simulink model "InvertedPD"  (Simulink 5.0)
settings: Solver=ode1  SolverMode=SingleTasking  StartTime=0.0  StopTime=70.0  FixedStep=0.001  RelTol=1e-3
libraries: pci1711 x3
CloseFcn:
  | rtwprivate ssgencode ModelCloseRequest InvertedPD
settings Model: LastModifiedBy=AD  ExtModeMexFile=rtwinext  ExtModeTrigMode=oneshot  ExtModeTrigDuration=100000  ExtModeLogAll=off  SimulationMode=external  LimitDataPoints=off  BlockReductionOpt=off  BooleanDataType=off  RTWSystemTargetFile=rtwinfbk.tlc  RTWTemplateMakefile=winfbktmf  RTWOptions="-aCCOptimize=1 -aEnforceIntegerDowncast=1 -aExtMode=1 -aFoldNonRolledExpr=1 -aForceParamTrailComments=0 -aGenerateComments=1 -aGenerateReport=0 -aIncDataTypeInIds=0 -aIncHierarchyInIds=0 -aInlineInvariantSignals=0 -aInlineParameters=0 -aInlinedPrmAccess=\"Literals\" -aLocalBlockOutputs=1 -aMaxRTWIdLen=31 -aPrefixModelToSubsysFcnNames=1 -aRTWVerbose=1 -aRebuildAll=0 -aRollThreshold=5 -aShowEliminatedStatements=1"

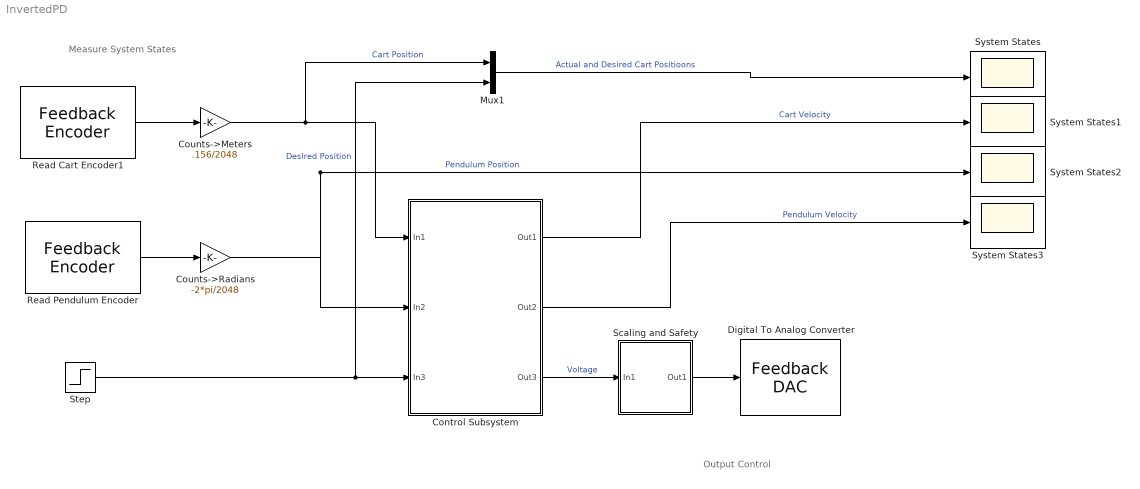
== system InvertedPD ==
  note: Measure System States
  note: Output Control
  Control Subsystem : Subsystem
  Counts->Meters : Gain  Gain=.156/2048  SaturateOnIntegerOverflow=on
  Counts->Radians : Gain  Gain=-2*pi/2048  SaturateOnIntegerOverflow=on
  Digital To Analog Converter : pci1711/Advantech  PCI1711 I//O Board Lib/Feedback DAC  channel=0  range=0  tsamp=0.001  hwAccess=on
  Mux1 : Mux  Inputs=2
  Read Cart Encoder1 : pci1711/Advantech  PCI1711 I//O Board Lib/Feedback Encoder   channel=0  offset=0  tsamp=0.001  hwAccess=on
  Read Pendulum Encoder : pci1711/Advantech  PCI1711 I//O Board Lib/Feedback Encoder   channel=1  offset=-1024  tsamp=0.001  hwAccess=on
  Scaling and Safety : Subsystem
  Step : Step  Time=20  After=0.2  SampleTime=0
  System States{,1..3} (4 alike) : Scope
      System States settings: TimeRange=50  YMin=-0.125  YMax=0.025  SaveName=y  Decimation=0.1  SampleInput=on  SampleTime=0.01
      System States1 settings: TimeRange=50  YMin=-0.125  YMax=0.025  SaveName=y1  Decimation=0.1  SampleInput=on  SampleTime=0.01
      System States2 settings: TimeRange=50  YMin=-0.125  YMax=0.025  SaveName=y2  Decimation=0.1  SampleInput=on  SampleTime=0.01
      System States3 settings: TimeRange=50  YMin=-0.125  YMax=0.025  SaveName=y3  Decimation=0.1  SampleInput=on  SampleTime=0.01
  wires:
  Counts->Meters/1 -> Mux1/1, Control Subsystem/1(In1)  "Cart Position"
  Counts->Radians/1 -> Control Subsystem/2(In2), System States2/1  "Pendulum Position"
  Scaling and Safety/1(Out1) -> Digital To Analog Converter/1
  Step/1 -> Mux1/2, Control Subsystem/3(In3)  "Desired Position"
  Control Subsystem/3(Out3) -> Scaling and Safety/1(In1)  "Voltage"
  Mux1/1 -> System States/1  "Actual and Desired Cart Positioons"
  Read Cart Encoder1/1 -> Counts->Meters/1
  Read Pendulum Encoder/1 -> Counts->Radians/1
  Control Subsystem/1(Out1) -> System States1/1  "Cart Velocity"
  Control Subsystem/2(Out2) -> System States3/1  "Pendulum Velocity"

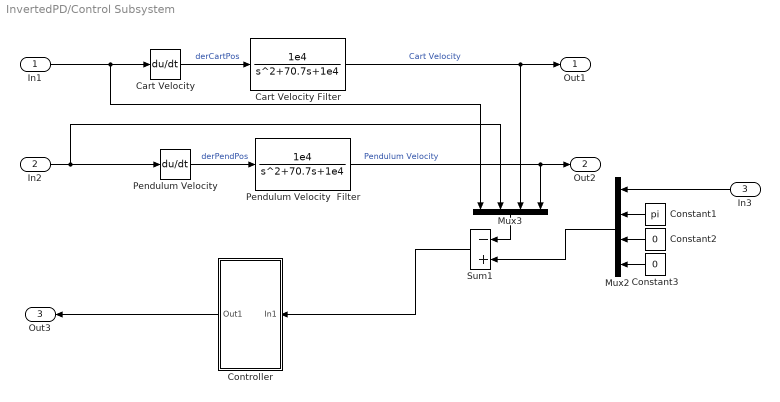
== system InvertedPD/Control Subsystem ==
  In1 : Inport
  In2 : Inport  Port=2
  In3 : Inport  Orientation=left  Port=3
  Cart Velocity : Derivative
  Cart Velocity Filter : TransferFcn  Numerator=[1e4]  Denominator=[1 70.7 1e4]
  Constant1 : Constant  Orientation=left  Value=pi
  Constant2 : Constant  Orientation=left  Value=0
  Constant3 : Constant  Orientation=left  Value=0
  Controller : Subsystem  Orientation=left
  Mux2 : Mux  Orientation=left
  Mux3 : Mux  Orientation=down
  Pendulum Velocity : Derivative
  Pendulum Velocity  Filter : TransferFcn  Numerator=[1e4]  Denominator=[1 70.7 1e4]
  Sum1 : Sum  Orientation=left  Inputs=-+  SaturateOnIntegerOverflow=on  InputSameDT=on
  Out1 : Outport
  Out2 : Outport  Port=2
  Out3 : Outport  Orientation=left  Port=3
  wires:
  Cart Velocity/1 -> Cart Velocity Filter/1  "derCartPos"
  Pendulum Velocity/1 -> Pendulum Velocity  Filter/1  "derPendPos"
  Cart Velocity Filter/1 -> Mux3/3, Out1/1  "Cart Velocity"
  Pendulum Velocity  Filter/1 -> Mux3/4, Out2/1  "Pendulum Velocity"
  Mux2/1 -> Sum1/2
  Constant1/1 -> Mux2/2
  Constant2/1 -> Mux2/3
  Constant3/1 -> Mux2/4
  Mux3/1 -> Sum1/1
  In1/1 -> Cart Velocity/1, Mux3/1
  In2/1 -> Pendulum Velocity/1, Mux3/2
  In3/1 -> Mux2/1
  Controller/1(Out1) -> Out3/1
  Sum1/1 -> Controller/1(In1)

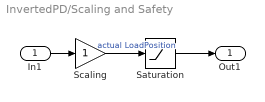
== system InvertedPD/Scaling and Safety ==
  In1 : Inport
  Saturation : Saturate  UpperLimit=2.5  LowerLimit=-2.5
  Scaling : Gain  SaturateOnIntegerOverflow=on
  Out1 : Outport
  wires:
  Saturation/1 -> Out1/1
  In1/1 -> Scaling/1
  Scaling/1 -> Saturation/1  "actual LoadPosition"

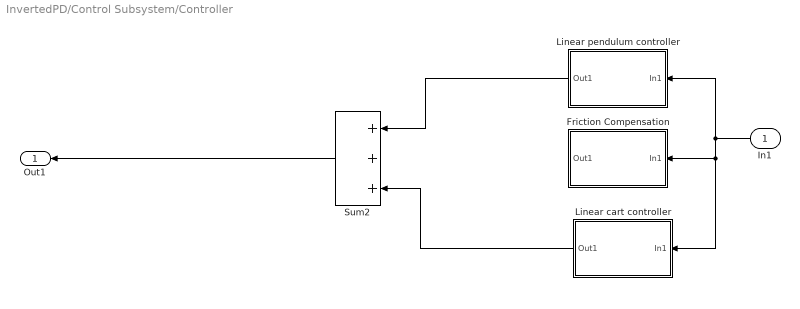
== system InvertedPD/Control Subsystem/Controller ==
  In1 : Inport  Orientation=left
  Friction Compensation : Subsystem  Orientation=left  mask(linear){frictionCompNeg=.1, frictionCompPos=.1}
      mask prompts: frictionCompNeg "Friction Compensation Magnitude in Negative Direction"; frictionCompPos "Friction Compensation Magnitude in Positive Direction"
      mask Display: plot(0,0,100,100,[40,30,20],[87,85,80],[46,54,54,46,46],[90,90,80,80,90],[46,45,45,46,54,55,55,54,46],[78,80,90,91,91,90,80,78,78],[51,51,49,49],[78,10,10,78],[90,80,70,60],[70,80,85,88],[20,10],[80,70],[20,20,15],[73,80,80],[85,80,80],[80,80,74])
  Linear cart controller : Subsystem  Orientation=left  mask(linear){K1=-40, K3=-80}
      mask prompts: K1 "K1  - position  feedback"; K3 "K3  -  velocity  feedback"
      mask Display: plot(0,0,100,100,[40,30,20],[87,85,80],[46,54,54,46,46],[90,90,80,80,90],[46,45,45,46,54,55,55,54,46],[78,80,90,91,91,90,80,78,78],[51,51,49,49],[78,10,10,78],[90,80,70,60],[70,80,85,88],[20,10],[80,70],[20,20,15],[73,80,80],[85,80,80],[80,80,74])
  Linear pendulum controller : Subsystem  Orientation=left  mask(linear){K2=130, K4=35}
      mask prompts: K2 "K2  - angle  feedback"; K4 "K4  - angular velocity  feedback"
      mask Display: plot(0,0,100,100,[40,30,20],[87,85,80],[46,54,54,46,46],[90,90,80,80,90],[46,45,45,46,54,55,55,54,46],[78,80,90,91,91,90,80,78,78],[51,51,49,49],[78,10,10,78],[90,80,70,60],[70,80,85,88],[20,10],[80,70],[20,20,15],[73,80,80],[85,80,80],[80,80,74])
  Sum2 : Sum  Orientation=left  Inputs=+++  SaturateOnIntegerOverflow=on  InputSameDT=on
  Out1 : Outport  Orientation=left
  wires:
  Linear pendulum controller/1(Out1) -> Sum2/1
  Linear cart controller/1(Out1) -> Sum2/3
  Sum2/1 -> Out1/1
  In1/1 -> Linear pendulum controller/1(In1), Friction Compensation/1(In1), Linear cart controller/1(In1)

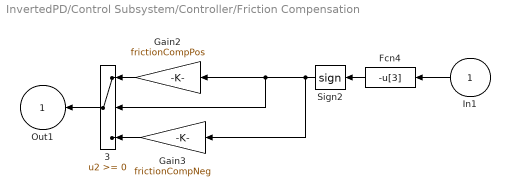
== system InvertedPD/Control Subsystem/Controller/Friction Compensation ==
  In1 : Inport  Orientation=left
  3 : Switch  Orientation=left  SaturateOnIntegerOverflow=on  InputSameDT=on
  Fcn4 : Fcn  Orientation=left  Expr=-u[3]
  Gain2 : Gain  Orientation=left  Gain=frictionCompPos  SaturateOnIntegerOverflow=on
  Gain3 : Gain  Orientation=left  Gain=frictionCompNeg  SaturateOnIntegerOverflow=on
  Sign2 : Signum  Tag=T  Orientation=left
  Out1 : Outport  Orientation=left  InitialOutput=0
  wires:
  Fcn4/1 -> Sign2/1
  In1/1 -> Fcn4/1
  Gain2/1 -> 3/1
  Gain3/1 -> 3/3
  Sign2/1 -> Gain3/1, Gain2/1, 3/2
  3/1 -> Out1/1

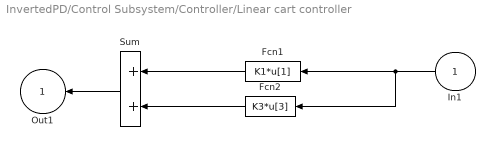
== system InvertedPD/Control Subsystem/Controller/Linear cart controller ==
  In1 : Inport  Orientation=left
  Fcn1 : Fcn  Orientation=left  Expr=K1*u[1]
  Fcn2 : Fcn  Orientation=left  Expr=K3*u[3]
  Sum : Sum  Orientation=left  SaturateOnIntegerOverflow=on  InputSameDT=on
  Out1 : Outport  Orientation=left  InitialOutput=0
  wires:
  Fcn1/1 -> Sum/1
  Fcn2/1 -> Sum/2
  Sum/1 -> Out1/1
  In1/1 -> Fcn1/1, Fcn2/1

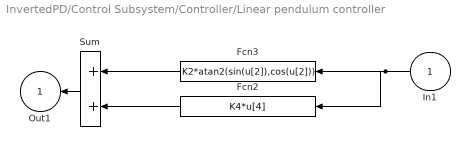
== system InvertedPD/Control Subsystem/Controller/Linear pendulum controller ==
  In1 : Inport  Orientation=left
  Fcn2 : Fcn  Orientation=left  Expr=K4*u[4]
  Fcn3 : Fcn  Orientation=left  Expr=K2*atan2(sin(u[2]),cos(u[2]))
  Sum : Sum  Orientation=left  SaturateOnIntegerOverflow=on  InputSameDT=on
  Out1 : Outport  Orientation=left  InitialOutput=0
  wires:
  Sum/1 -> Out1/1
  Fcn2/1 -> Sum/2
  In1/1 -> Fcn2/1, Fcn3/1
  Fcn3/1 -> Sum/1
